simulink model "FingerEAERCtrl"  (R2012b)
settings: Solver=ode3  StartTime=0.0  StopTime=inf  FixedStep=.001  RelTol=1e-3
PreLoadFcn:
  | settupFilter;
InitFcn:
  | settupFilter;
values from neighbouring files (symbols this model uses):
  x0low = (eye(size(Alow))-Alow)\Blow*0    [settupFilter.m]
undefined symbols (not defined in the file or in its folder): Alow, Blow, Clow, Dlow
libraries: xpcnilib x4, xpclib x4, simulink x2
(part 1 of 2)
settings Model: SimulationMode=external  BufferReuse=off  Creator=Admin  LastModifiedBy=Admin
settings OptimizationCC: BlockReduction=off  OptimizeBlockIOStorage=off  BufferReuse=off  ExpressionFolding=off  LocalBlockOutputs=off
settings HardwareCC: ProdIntDivRoundTo=Zero  ProdEndianess=LittleEndian  ProdHWDeviceType=Generic->32-bit x86 compatible
settings RTWCC: SystemTargetFile=xpctarget.tlc  TemplateMakefile=xpc_default_tmf  Description=xPC Target  ProcessScript=xpctarget_make_rtw_hook  RTWCompilerOptimization=On
settings xpcTargetCC: TargetFcnLib=ansi_tfl_table_tmw.mat  CodeReplacementLibrary=XPC_BLAS  ParMdlRefBuildCompliant=on  ConcurrentExecutionCompliant=on  CombineSignalStateStructs=off  GRTInterface=on  xPCTaskExecutionProfile=off  xPCRL32EventNumber=5000  xPCLoadParamSetFile=off  xPCConcurrentTasks=off  xPCEnableSFAnimation=off

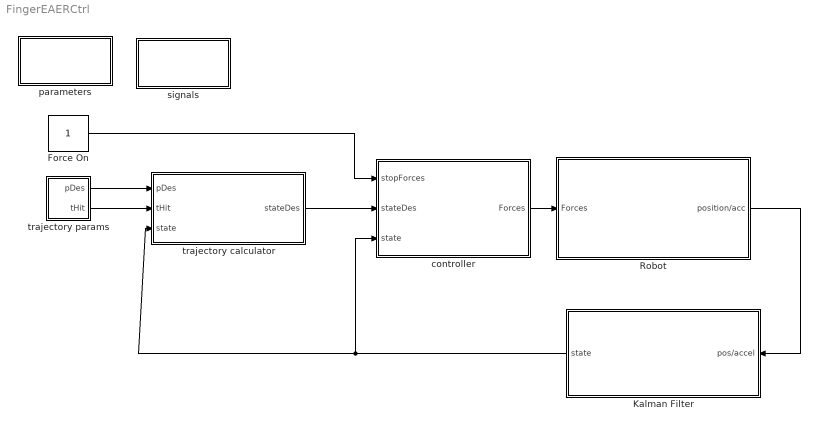
== system FingerEAERCtrl ==
  Force On : Constant
  Kalman Filter : Subsystem
  Robot : Subsystem
  controller : Subsystem
  parameters : Subsystem
  signals : Subsystem
  trajectory calculator : Subsystem
  trajectory params : Subsystem
  wires:
  Robot/1(position/acc) -> Kalman Filter/1(pos/accel)
  trajectory calculator/1(stateDes) -> controller/2(stateDes)
  controller/1(Forces) -> Robot/1(Forces)
  Kalman Filter/1(state) -> trajectory calculator/3(state), controller/3(state)
  trajectory params/1(pDes) -> trajectory calculator/1(pDes)
  trajectory params/2(tHit) -> trajectory calculator/2(tHit)
  Force On/1 -> controller/1(stopForces)

== system FingerEAERCtrl/Kalman Filter ==
  pos/accel : Inport
  Demux : Demux
  Mux : Mux  Inputs=2
  kalman1 : Subsystem
  kalman2 : Subsystem
  state : Outport
  tag scope: SIG_STATE=global
  wires:
  Demux/1 -> kalman1/1(position)
  Demux/2 -> kalman2/1(position)
  Demux/3 -> kalman1/2(acc)
  Demux/4 -> kalman2/2(acc)
  pos/accel/1 -> Demux/1
  kalman1/1(position/est_vel) -> Mux/1
  kalman2/1(position/est_vel) -> Mux/2
  Mux/1 -> [SIG_STATE], state/1

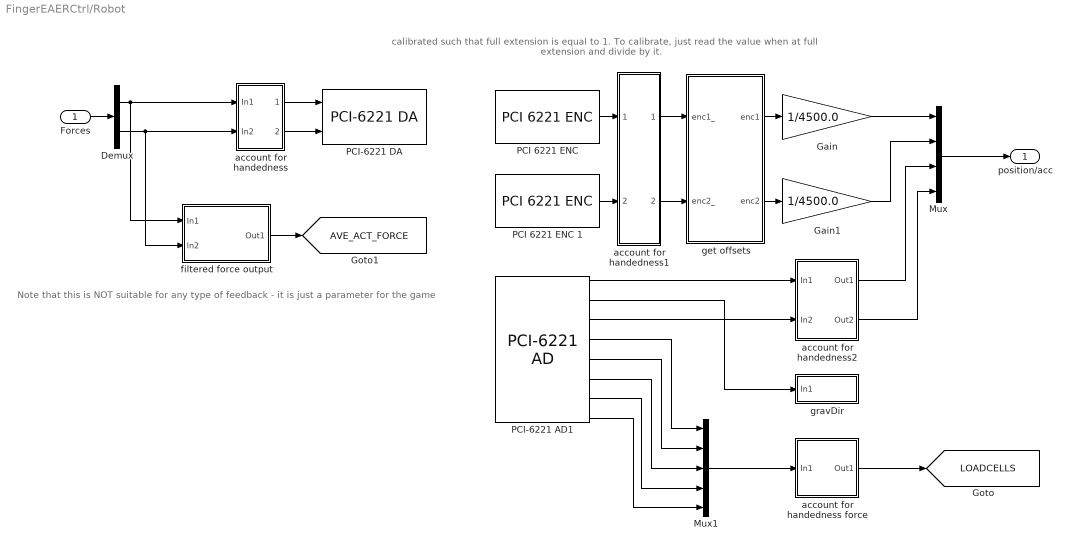
== system FingerEAERCtrl/Robot ==
  note: Note that this is NOT suitable for any type
      | of feedback - it is just a parameter for the game
  note: calibrated such that full extension is equal to 1. To calibrate, just read the value when at full extension and divide by it.
  Forces : Inport
  Demux : Demux  Outputs=2
  Gain : Gain  Gain=1/4500.0
  Gain1 : Gain  Gain=1/4500.0
  Mux : Mux
  Mux1 : Mux  Inputs=5
  "PCI 6221 ENC " : xpcnilib/Incremental Encoder/PCI 6221 ENC   channel=0  countMode=Quadrature Mode x4  initCount=0  reload=off  indexPhase=A low B low  filter=Minimum pulse width 125 nanoseconds  sampleTime=0.001  slot=-1
  PCI 6221 ENC 1 : xpcnilib/Incremental Encoder/PCI 6221 ENC   channel=1  countMode=Quadrature Mode x4  initCount=0  reload=off  indexPhase=A low B low  filter=Minimum pulse width 125 nanoseconds  sampleTime=0.001  slot=-1
  PCI-6221 AD1 : xpcnilib/A//D/M Series/PCI-6221 AD  channel=[1 2 3 4 5 6 7 8]  range=[10]  coupling=[0]  scantime=5e-6  sampletime=0.001  slot=-1
  PCI-6221 DA : xpcnilib/D//A/M Series/PCI-6221 DA  channel=[1 2]  reset=[1]  initValue=[0]  sampletime=0.001  slot=-1
  account for handedness : Subsystem
  account for handedness force : Subsystem
  account for handedness1 : Subsystem
  account for handedness2 : Subsystem
  filtered force output : Subsystem
  get offsets : Subsystem
  gravDir : Subsystem
  position/acc : Outport
  tag scope: AVE_ACT_FORCE=global, LOADCELLS=global
  wires:
  Gain/1 -> Mux/1
  Mux/1 -> position/acc/1
  Forces/1 -> Demux/1
  Gain1/1 -> Mux/2
  get offsets/1(enc1) -> Gain/1
  get offsets/2(enc2) -> Gain1/1
  Demux/1 -> filtered force output/1(In1), account for handedness/1(In1)
  Demux/2 -> filtered force output/2(In2), account for handedness/2(In2)
  account for handedness/2(Out2) -> PCI-6221 DA/2
  account for handedness/1(Out1) -> PCI-6221 DA/1
  "PCI 6221 ENC "/1 -> account for handedness1/1(In1)
  account for handedness1/1(Out1) -> get offsets/1(enc1_)
  account for handedness1/2(Out2) -> get offsets/2(enc2_)
  PCI 6221 ENC 1/1 -> account for handedness1/2(In2)
  PCI-6221 AD1/1 -> account for handedness2/1(In1)
  PCI-6221 AD1/3 -> account for handedness2/2(In2)
  account for handedness2/1(Out1) -> Mux/3
  account for handedness2/2(Out2) -> Mux/4
  PCI-6221 AD1/4 -> Mux1/1
  PCI-6221 AD1/5 -> Mux1/2
  PCI-6221 AD1/6 -> Mux1/3
  PCI-6221 AD1/7 -> Mux1/4
  PCI-6221 AD1/8 -> Mux1/5
  Mux1/1 -> account for handedness force/1(In1)
  account for handedness force/1(Out1) -> [LOADCELLS]
  PCI-6221 AD1/2 -> gravDir/1(In1)
  filtered force output/1(Out1) -> [AVE_ACT_FORCE]

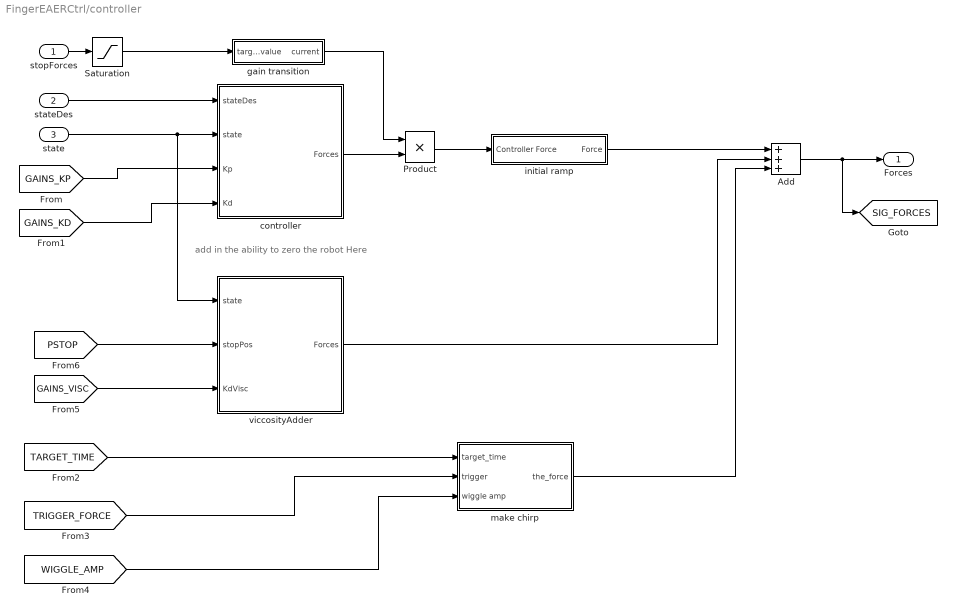
== system FingerEAERCtrl/controller ==
  note: add in the ability to zero the robot Here
  stopForces : Inport
  stateDes : Inport  Port=2
  state : Inport  Port=3
  Add : Sum  Inputs=+++
  Product : Product  RndMeth=Zero
  Saturation : Saturate  UpperLimit=1  LowerLimit=0
  controller : MATLAB Function  TreatAsAtomicUnit=on
  gain transition : Subsystem
  initial ramp : Subsystem
  make chirp : Subsystem
  viccosityAdder : MATLAB Function  TreatAsAtomicUnit=on
  Forces : Outport
  tag scope: SIG_FORCES=global
  wires:
  state/1 -> viccosityAdder/1(state), controller/2(state)
  [GAINS_KD] -> controller/4(Kd)
  [GAINS_KP] -> controller/3(Kp)
  stateDes/1 -> controller/1(stateDes)
  stopForces/1 -> Saturation/1
  Saturation/1 -> gain transition/1(target_value)
  controller/1(Forces) -> Product/2
  gain transition/1(current) -> Product/1
  Product/1 -> initial ramp/1(Controller Force)
  initial ramp/1(Force) -> Add/1
  Add/1 -> [SIG_FORCES], Forces/1
  [TARGET_TIME] -> make chirp/1(target_time)
  [TRIGGER_FORCE] -> make chirp/2(trigger)
  make chirp/1(the_force) -> Add/3
  [WIGGLE_AMP] -> make chirp/3(wiggle amp)
  viccosityAdder/1(Forces) -> Add/2
  [GAINS_VISC] -> viccosityAdder/3(KdVisc)
  [PSTOP] -> viccosityAdder/2(stopPos)

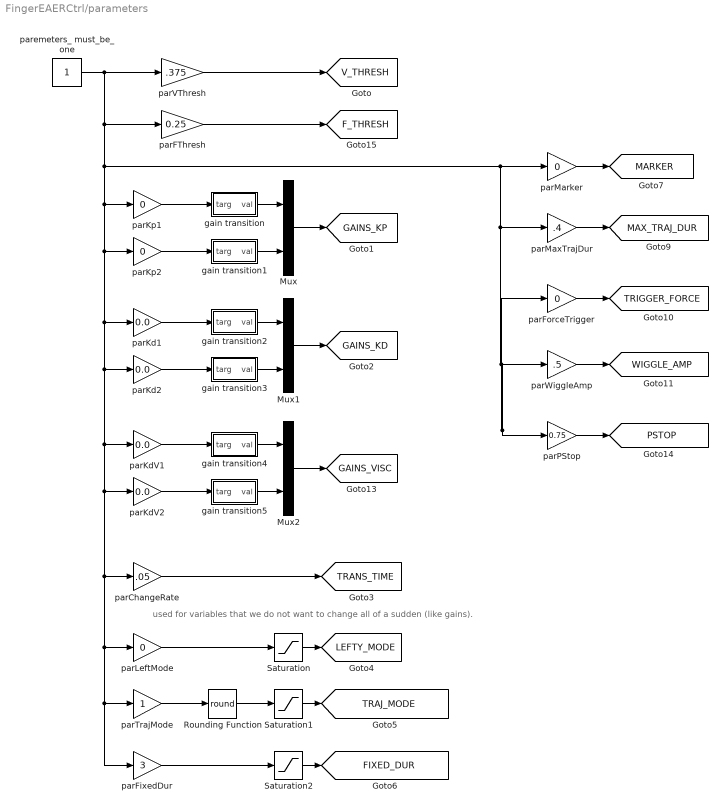
== system FingerEAERCtrl/parameters ==
  note: used for variables that we do not want to change all of a sudden (like gains).
  Mux : Mux  Inputs=2
  Mux1 : Mux  Inputs=2
  Mux2 : Mux  Inputs=2
  Rounding Function : Rounding  Operator=round
  Saturation : Saturate  UpperLimit=1  LowerLimit=0
  Saturation1 : Saturate  UpperLimit=4  LowerLimit=1
  Saturation2 : Saturate  UpperLimit=10  LowerLimit=.25
  gain transition : Subsystem
  gain transition1 : Subsystem
  gain transition2 : Subsystem
  gain transition3 : Subsystem
  gain transition4 : Subsystem
  gain transition5 : Subsystem
  parChangeRate : Gain  Gain=.05
  parFThresh : Gain  Gain=0.25
  parFixedDur : Gain  Gain=3
  parForceTrigger : Gain  Gain=0
  parKd1 : Gain  Gain=0.0
  parKd2 : Gain  Gain=0.0
  parKdV1 : Gain  Gain=0.0
  parKdV2 : Gain  Gain=0.0
  parKp1 : Gain  Gain=0
  parKp2 : Gain  Gain=0
  parLeftMode : Gain  Gain=0
  parMarker : Gain  Gain=0
  parMaxTrajDur : Gain  Gain=.4
  parPStop : Gain  Gain=0.75
  parTrajMode : Gain
  parVThresh : Gain  Gain=.375
  parWiggleAmp : Gain  Gain=.5
  paremeters_ must_be_one : Constant
  tag scope: FIXED_DUR=global, F_THRESH=global, GAINS_KD=global, GAINS_KP=global, GAINS_VISC=global, LEFTY_MODE=global, MARKER=global, MAX_TRAJ_DUR=global, PSTOP=global, TRAJ_MODE=global, TRANS_TIME=global, TRIGGER_FORCE=global, V_THRESH=global, WIGGLE_AMP=global
  wires:
  Mux/1 -> [GAINS_KP]
  Mux1/1 -> [GAINS_KD]
  Saturation/1 -> [LEFTY_MODE]
  gain transition/1(val) -> Mux/1
  gain transition1/1(val) -> Mux/2
  gain transition2/1(val) -> Mux1/1
  gain transition3/1(val) -> Mux1/2
  parVThresh/1 -> [V_THRESH]
  parKp1/1 -> gain transition/1(targ)
  parKp2/1 -> gain transition1/1(targ)
  parKd1/1 -> gain transition2/1(targ)
  parKd2/1 -> gain transition3/1(targ)
  parChangeRate/1 -> [TRANS_TIME]
  parLeftMode/1 -> Saturation/1
  Saturation1/1 -> [TRAJ_MODE]
  parTrajMode/1 -> Rounding Function/1
  Saturation2/1 -> [FIXED_DUR]
  parFixedDur/1 -> Saturation2/1
  Rounding Function/1 -> Saturation1/1
  parMarker/1 -> [MARKER]
  parMaxTrajDur/1 -> [MAX_TRAJ_DUR]
  parForceTrigger/1 -> [TRIGGER_FORCE]
  parWiggleAmp/1 -> [WIGGLE_AMP]
  Mux2/1 -> [GAINS_VISC]
  gain transition4/1(val) -> Mux2/1
  gain transition5/1(val) -> Mux2/2
  parKdV1/1 -> gain transition4/1(targ)
  parKdV2/1 -> gain transition5/1(targ)
  paremeters_ must_be_one/1 -> parVThresh/1, parFThresh/1, parKp1/1, parKp2/1, parKd1/1, parKd2/1, parKdV1/1, parKdV2/1, parChangeRate/1, parLeftMode/1, parFixedDur/1, parTrajMode/1, parPStop/1, parWiggleAmp/1, parForceTrigger/1, parMaxTrajDur/1, parMarker/1
  parPStop/1 -> [PSTOP]
  parFThresh/1 -> [F_THRESH]

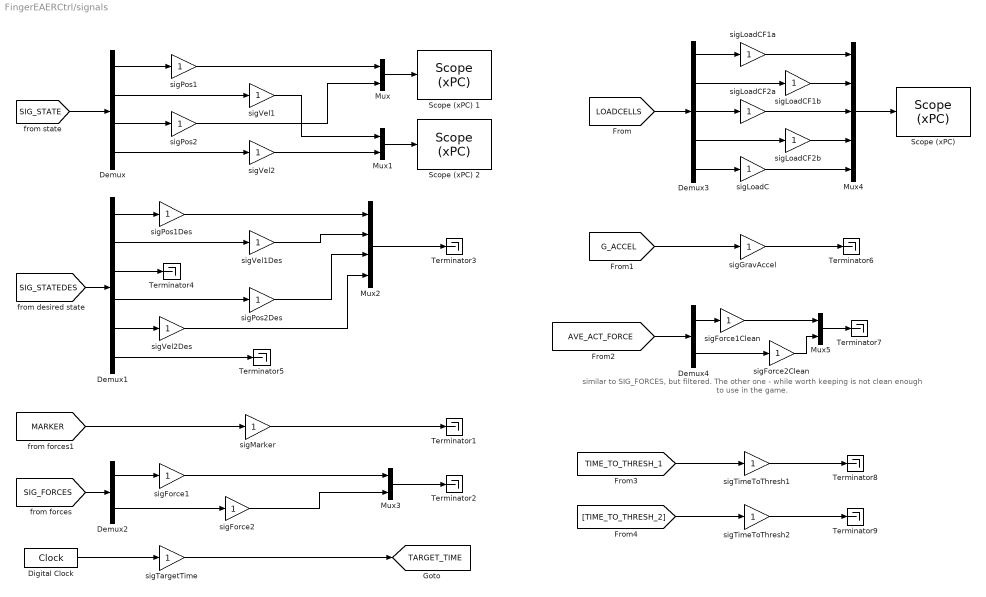
== system FingerEAERCtrl/signals ==
  note: similar to SIG_FORCES, but filtered. The other one - while worth keeping is not clean enough to use in the game.
  Demux : Demux
  Demux1 : Demux  Outputs=6
  Demux2 : Demux  Outputs=2
  Demux3 : Demux  Outputs=5
  Demux4 : Demux  Outputs=2
  Digital Clock : DigitalClock  SampleTime=.001
  Mux{,1,3,5} (4 alike) : Mux  Inputs=2
  Mux2 : Mux
  Mux4 : Mux  Inputs=5
  "Scope (xPC) " : xpclib/Misc./Scope (xPC)   scopeno=5  scopetype=Target  autostart=on  viewmode=Graphical redraw  formatstr='%15.6f'  grid=on  ylimits=[-3,3]  nosamples=500  noprepostsamples=0  interleave=1  triggermode=FreeRun  triggersignal=1  triggerlevel=0.0  triggerslope=Either  triggerscope=1  triggersample=0  filename=data.dat  mode=Lazy  writesize=512  autorestart=off  dynamicfilemode=off  maxwritefilesize=512*1024^2
  Scope (xPC) 1 : xpclib/Misc./Scope (xPC)   scopeno=1  scopetype=Target  autostart=on  viewmode=Graphical redraw  formatstr='%15.6f'  grid=on  ylimits=[0,1.1]  nosamples=500  noprepostsamples=0  interleave=1  triggermode=FreeRun  triggersignal=1  triggerlevel=0.0  triggerslope=Either  triggerscope=1  triggersample=0  filename=data.dat  mode=Lazy  writesize=512  autorestart=off  dynamicfilemode=off  maxwritefilesize=512*1024^2
  Scope (xPC) 2 : xpclib/Misc./Scope (xPC)   scopeno=2  scopetype=Target  autostart=on  viewmode=Graphical redraw  formatstr='%15.6f'  grid=on  ylimits=[-10,10]  nosamples=500  noprepostsamples=0  interleave=1  triggermode=FreeRun  triggersignal=1  triggerlevel=0.0  triggerslope=Either  triggerscope=1  triggersample=0  filename=data.dat  mode=Lazy  writesize=512  autorestart=off  dynamicfilemode=off  maxwritefilesize=512*1024^2
  Terminator{1..9} (9 alike) : Terminator
  sigForce1 : Gain
  sigForce1Clean : Gain
  sigForce2 : Gain
  sigForce2Clean : Gain
  sigGravAccel : Gain
  sigLoadC : Gain
  sigLoadCF1a : Gain
  sigLoadCF1b : Gain
  sigLoadCF2a : Gain
  sigLoadCF2b : Gain
  sigMarker : Gain
  sigPos1 : Gain
  sigPos1Des : Gain
  sigPos2 : Gain
  sigPos2Des : Gain
  sigTargetTime : Gain
  sigTimeToThresh1 : Gain
  sigTimeToThresh2 : Gain
  sigVel1 : Gain
  sigVel1Des : Gain
  sigVel2 : Gain
  sigVel2Des : Gain
  tag scope: TARGET_TIME=global
  wires:
  [SIG_STATE] -> Demux/1
  Demux/1 -> sigPos1/1
  Demux/2 -> sigVel1/1
  Demux/3 -> sigPos2/1
  Demux/4 -> sigVel2/1
  [SIG_STATEDES] -> Demux1/1
  Demux1/1 -> sigPos1Des/1
  Demux1/2 -> sigVel1Des/1
  Demux1/3 -> Terminator4/1
  Demux1/4 -> sigPos2Des/1
  Demux1/5 -> sigVel2Des/1
  Demux1/6 -> Terminator5/1
  Mux/1 -> Scope (xPC) 1/1
  Mux1/1 -> Scope (xPC) 2/1
  sigPos1/1 -> Mux/1
  sigPos2/1 -> Mux/2
  sigVel1/1 -> Mux1/1
  sigVel2/1 -> Mux1/2
  sigPos1Des/1 -> Mux2/1
  sigVel1Des/1 -> Mux2/2
  sigPos2Des/1 -> Mux2/3
  sigVel2Des/1 -> Mux2/4
  Mux2/1 -> Terminator3/1
  [SIG_FORCES] -> Demux2/1
  Demux2/1 -> sigForce1/1
  Demux2/2 -> sigForce2/1
  Mux3/1 -> Terminator2/1
  sigForce1/1 -> Mux3/1
  sigForce2/1 -> Mux3/2
  Digital Clock/1 -> sigTargetTime/1
  sigTargetTime/1 -> [TARGET_TIME]
  [MARKER] -> sigMarker/1
  sigMarker/1 -> Terminator1/1
  [LOADCELLS] -> Demux3/1
  Demux3/1 -> sigLoadCF1a/1
  Demux3/2 -> sigLoadCF1b/1
  Demux3/3 -> sigLoadCF2a/1
  Demux3/4 -> sigLoadCF2b/1
  Demux3/5 -> sigLoadC/1
  sigLoadCF1a/1 -> Mux4/1
  sigLoadCF1b/1 -> Mux4/2
  sigLoadCF2a/1 -> Mux4/3
  sigLoadCF2b/1 -> Mux4/4
  sigLoadC/1 -> Mux4/5
  Mux4/1 -> "Scope (xPC) "/1
  [G_ACCEL] -> sigGravAccel/1
  sigGravAccel/1 -> Terminator6/1
  [AVE_ACT_FORCE] -> Demux4/1
  Demux4/1 -> sigForce1Clean/1
  Demux4/2 -> sigForce2Clean/1
  Mux5/1 -> Terminator7/1
  sigForce1Clean/1 -> Mux5/1
  sigForce2Clean/1 -> Mux5/2
  sigTimeToThresh1/1 -> Terminator8/1
  [TIME_TO_THRESH_1] -> sigTimeToThresh1/1
  sigTimeToThresh2/1 -> Terminator9/1
  [TIME_TO_THRESH_2] -> sigTimeToThresh2/1

== system FingerEAERCtrl/trajectory calculator ==
  pDes : Inport
  tHit : Inport  Port=2
  state : Inport  Port=3
  Multiport Switch : MultiPortSwitch  Inputs=4
  mode 1: sub-init : Subsystem
  mode 2: auto initiated : Subsystem
  mode 3: auto init no return : Subsystem
  mode 4: sub init no return : Subsystem
  stateDes : Outport
  tag scope: SIG_STATEDES=global
  wires:
  pDes/1 -> mode 4: sub init no return/1(pDes), mode 3: auto init no return/1(pDes), mode 2: auto initiated/1(pDes), mode 1: sub-init/1(pDes)
  state/1 -> mode 1: sub-init/3(state), mode 4: sub init no return/3(state), mode 3: auto init no return/3(state), mode 2: auto initiated/3(state)
  mode 1: sub-init/1(trajectory) -> Multiport Switch/2
  mode 2: auto initiated/1(trajectory) -> Multiport Switch/3
  mode 3: auto init no return/1(trajectory) -> Multiport Switch/4
  [TRAJ_MODE] -> Multiport Switch/1
  mode 4: sub init no return/1(trajectory) -> Multiport Switch/5
  Multiport Switch/1 -> [SIG_STATEDES], stateDes/1
  tHit/1 -> mode 4: sub init no return/2(tHit), mode 3: auto init no return/2(tHit), mode 2: auto initiated/2(tHit), mode 1: sub-init/2(tHit)

== system FingerEAERCtrl/trajectory params ==
  Mux : Mux  Inputs=2
  Mux1 : Mux  Inputs=2
  parP1Des : Gain  Gain=.95
  parP2Des : Gain  Gain=.95
  parTHit1 : Gain  Gain=50
  parTHit2 : Gain  Gain=40
  unity_traj : Constant
  pDes : Outport
  tHit : Outport  Port=2
  wires:
  Mux/1 -> pDes/1
  Mux1/1 -> tHit/1
  parP1Des/1 -> Mux/1
  parP2Des/1 -> Mux/2
  parTHit1/1 -> Mux1/1
  parTHit2/1 -> Mux1/2
  unity_traj/1 -> parTHit2/1, parTHit1/1, parP2Des/1, parP1Des/1

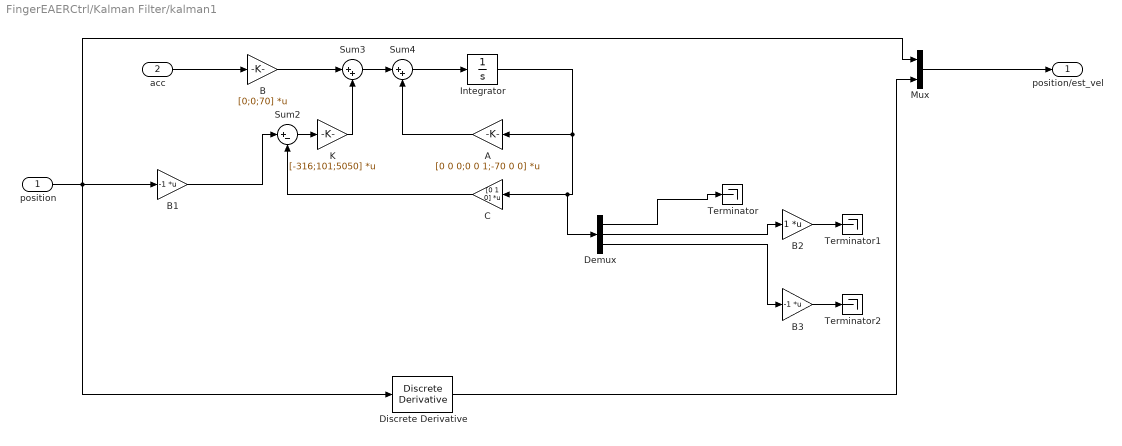
== system FingerEAERCtrl/Kalman Filter/kalman1 ==
  position : Inport
  acc : Inport  Port=2
  A : Gain  Gain=[0 0 0;0 0 1;-70 0 0]  Multiplication=Matrix(K*u)
  B : Gain  Gain=[0;0;70]  Multiplication=Matrix(K*u)
  B1 : Gain  Gain=-1  Multiplication=Matrix(K*u)
  B2 : Gain  Multiplication=Matrix(K*u)
  B3 : Gain  Gain=-1  Multiplication=Matrix(K*u)
  C : Gain  Gain=[0 1 0]  Multiplication=Matrix(K*u)
  Demux : Demux  Outputs=3
  Discrete Derivative : simulink/Discrete/Discrete Derivative  gainval=1.0  ICPrevScaledInput=0.0  InputProcessing=Inherited  OutMin=[]  OutMax=[]  OutDataType=fixdt(1, 16)  OutScaling=2^-10  DoSatur=off
  Integrator : Integrator  InitialCondition=[1.5;0;0]
  K : Gain  Gain=[-316;101;5050]  Multiplication=Matrix(K*u)
  Mux : Mux  Inputs=2
  Sum2 : Sum  Inputs=|+-
  Sum3 : Sum  Inputs=|++
  Sum4 : Sum  Inputs=|++
  Terminator : Terminator
  Terminator1 : Terminator
  Terminator2 : Terminator
  position/est_vel : Outport
  wires:
  Integrator/1 -> A/1, C/1, Demux/1
  C/1 -> Sum2/2
  Sum2/1 -> K/1
  B/1 -> Sum3/1
  K/1 -> Sum3/2
  Sum3/1 -> Sum4/1
  A/1 -> Sum4/2
  Sum4/1 -> Integrator/1
  Demux/2 -> B2/1
  Demux/3 -> B3/1
  Demux/1 -> Terminator/1
  B1/1 -> Sum2/1
  B2/1 -> Terminator1/1
  Mux/1 -> position/est_vel/1
  acc/1 -> B/1
  position/1 -> Discrete Derivative/1, Mux/1, B1/1
  Discrete Derivative/1 -> Mux/2
  B3/1 -> Terminator2/1

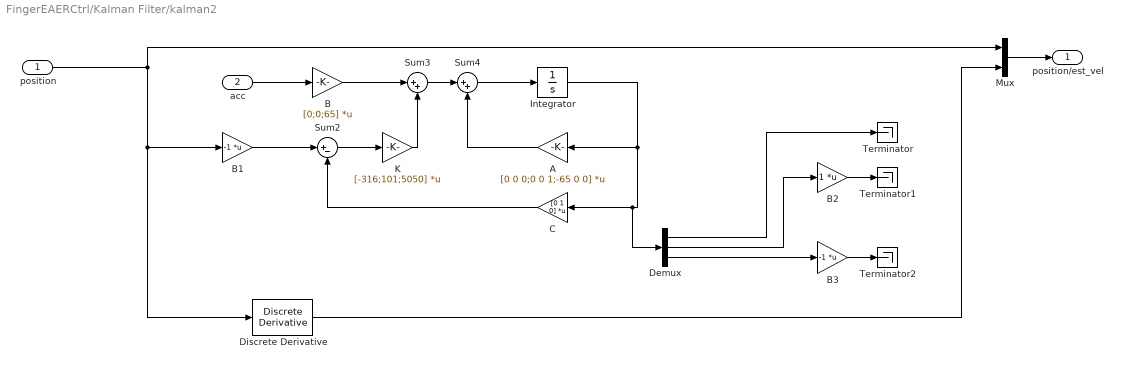
== system FingerEAERCtrl/Kalman Filter/kalman2 ==
  position : Inport
  acc : Inport  Port=2
  A : Gain  Gain=[0 0 0;0 0 1;-65 0 0]  Multiplication=Matrix(K*u)
  B : Gain  Gain=[0;0;65]  Multiplication=Matrix(K*u)
  B1 : Gain  Gain=-1  Multiplication=Matrix(K*u)
  B2 : Gain  Multiplication=Matrix(K*u)
  B3 : Gain  Gain=-1  Multiplication=Matrix(K*u)
  C : Gain  Gain=[0 1 0]  Multiplication=Matrix(K*u)
  Demux : Demux  Outputs=3
  Discrete Derivative : simulink/Discrete/Discrete Derivative  gainval=1.0  ICPrevScaledInput=0.0  InputProcessing=Inherited  OutMin=[]  OutMax=[]  OutDataType=fixdt(1, 16)  OutScaling=2^-10  DoSatur=off
  Integrator : Integrator  InitialCondition=[1.5;0;0]
  K : Gain  Gain=[-316;101;5050]  Multiplication=Matrix(K*u)
  Mux : Mux  Inputs=2
  Sum2 : Sum  Inputs=|+-
  Sum3 : Sum  Inputs=|++
  Sum4 : Sum  Inputs=|++
  Terminator : Terminator
  Terminator1 : Terminator
  Terminator2 : Terminator
  position/est_vel : Outport
  wires:
  acc/1 -> B/1
  Mux/1 -> position/est_vel/1
  B2/1 -> Terminator1/1
  B1/1 -> Sum2/1
  Demux/1 -> Terminator/1
  Demux/3 -> B3/1
  Demux/2 -> B2/1
  Sum4/1 -> Integrator/1
  A/1 -> Sum4/2
  Sum3/1 -> Sum4/1
  K/1 -> Sum3/2
  B/1 -> Sum3/1
  Sum2/1 -> K/1
  C/1 -> Sum2/2
  Integrator/1 -> Demux/1, C/1, A/1
  position/1 -> Discrete Derivative/1, B1/1, Mux/1
  Discrete Derivative/1 -> Mux/2
  B3/1 -> Terminator2/1

== system FingerEAERCtrl/Robot/account for handedness ==
  In1 : Inport
  In2 : Inport  Port=2
  MATLAB Function : MATLAB Function  TreatAsAtomicUnit=on
  Out1 : Outport
  Out2 : Outport  Port=2
  wires:
  MATLAB Function/1(output1) -> Out1/1
  MATLAB Function/2(output2) -> Out2/1
  In1/1 -> MATLAB Function/1(input1)
  In2/1 -> MATLAB Function/2(input2)
  [LEFTY_MODE] -> MATLAB Function/3(leftyMode)

== system FingerEAERCtrl/Robot/account for handedness force ==
  In1 : Inport
  MATLAB Function : MATLAB Function  TreatAsAtomicUnit=on
  Out1 : Outport
  wires:
  [LEFTY_MODE] -> MATLAB Function/2(leftyMode)
  MATLAB Function/1(output) -> Out1/1
  In1/1 -> MATLAB Function/1(inp1)

== system FingerEAERCtrl/Robot/account for handedness1 ==
  In1 : Inport
  In2 : Inport  Port=2
  MATLAB Function : MATLAB Function  TreatAsAtomicUnit=on
  Out1 : Outport
  Out2 : Outport  Port=2
  wires:
  MATLAB Function/1(output1) -> Out1/1
  MATLAB Function/2(output2) -> Out2/1
  In1/1 -> MATLAB Function/1(input1)
  In2/1 -> MATLAB Function/2(input2)
  [LEFTY_MODE] -> MATLAB Function/3(leftyMode)

== system FingerEAERCtrl/Robot/account for handedness2 ==
  In1 : Inport
  In2 : Inport  Port=2
  MATLAB Function : MATLAB Function  TreatAsAtomicUnit=on
  Out1 : Outport
  Out2 : Outport  Port=2
  wires:
  MATLAB Function/1(output1) -> Out1/1
  MATLAB Function/2(output2) -> Out2/1
  In1/1 -> MATLAB Function/1(input1)
  In2/1 -> MATLAB Function/2(input2)
  [LEFTY_MODE] -> MATLAB Function/3(leftyMode)

== system FingerEAERCtrl/Robot/filtered force output ==
  In1 : Inport
  In2 : Inport  Port=2
  Low Pass 100 Hz : DiscreteStateSpace  A=Alow  B=Blow  C=Clow  D=Dlow  X0=x0low  SampleTime=-1
  Low Pass 100 Hz1 : DiscreteStateSpace  A=Alow  B=Blow  C=Clow  D=Dlow  X0=x0low  SampleTime=-1
  Memory : Memory
  Memory1 : Memory
  Mux2 : Mux  Inputs=2
  Out1 : Outport
  wires:
  Low Pass 100 Hz1/1 -> Memory1/1
  Low Pass 100 Hz/1 -> Memory/1
  Mux2/1 -> Out1/1
  In1/1 -> Low Pass 100 Hz/1
  In2/1 -> Low Pass 100 Hz1/1
  Memory/1 -> Mux2/1
  Memory1/1 -> Mux2/2

== system FingerEAERCtrl/Robot/get offsets ==
  enc1_ : Inport
  enc2_ : Inport  Port=2
  Digital Clock : DigitalClock  SampleTime=.001
  MATLAB Function : MATLAB Function  TreatAsAtomicUnit=on
  Memory : Memory
  Memory1 : Memory  X0=[0,0]
  enc1 : Outport
  enc2 : Outport  Port=2
  wires:
  Memory/1 -> MATLAB Function/5(nSamples_)
  Memory1/1 -> MATLAB Function/4(summedVals_)
  MATLAB Function/3(summedVals) -> Memory1/1
  Digital Clock/1 -> MATLAB Function/3(time)
  MATLAB Function/1(encoder1) -> enc1/1
  MATLAB Function/2(encoder2) -> enc2/1
  enc2_/1 -> MATLAB Function/2(enc2_)
  enc1_/1 -> MATLAB Function/1(enc1_)
  MATLAB Function/4(nSamples) -> Memory/1

== system FingerEAERCtrl/Robot/gravDir ==
  In1 : Inport
  Constant : Constant  Value=1.5
  Scope (xPC) 1 : xpclib/Misc./Scope (xPC)   scopeno=3  scopetype=Target  autostart=on  viewmode=Graphical redraw  formatstr='%15.6f'  grid=on  ylimits=[.03,.1]  nosamples=500  noprepostsamples=0  interleave=1  triggermode=FreeRun  triggersignal=1  triggerlevel=0.0  triggerslope=Either  triggerscope=1  triggersample=0  filename=data.dat  mode=Lazy  writesize=512  autorestart=off  dynamicfilemode=off  maxwritefilesize=512*1024^2
  Sum : Sum  Inputs=|+-
  gain : Gain  Gain=.172
  tag scope: G_ACCEL=global
  wires:
  gain/1 -> [G_ACCEL], Scope (xPC) 1/1
  Sum/1 -> gain/1
  Constant/1 -> Sum/2
  In1/1 -> Sum/1

== system FingerEAERCtrl/controller/gain transition ==
  target_value : Inport
  Memory : Memory  X0=zeros(1,4)
  gainramp : MATLAB Function  TreatAsAtomicUnit=on
  current : Outport
  wires:
  Memory/1 -> gainramp/3(state)
  gainramp/2(state1) -> Memory/1
  [TRANS_TIME] -> gainramp/1(tr)
  gainramp/1(val) -> current/1
  target_value/1 -> gainramp/2(valD)

== system FingerEAERCtrl/controller/initial ramp ==
  note: In the first five seconds of operation, have the actuators pull the fingers back so that the robot can zero itself accurately
  Controller Force : Inport
  MATLAB Function : MATLAB Function  TreatAsAtomicUnit=on
  Saturation1 : Saturate  UpperLimit=2.5  LowerLimit=-2.5
  ramp : MATLAB Function  TreatAsAtomicUnit=on
  Force : Outport
  wires:
  ramp/1(y) -> Saturation1/1
  Controller Force/1 -> MATLAB Function/1(ctrlForce)
  Saturation1/1 -> MATLAB Function/2(rampForce)
  [TARGET_TIME] -> MATLAB Function/3(time), ramp/1(tTime)
  MATLAB Function/1(Force) -> Force/1

== system FingerEAERCtrl/controller/make chirp ==
  target_time : Inport
  trigger : Inport  Port=2
  wiggle amp : Inport  Port=3
  MATLAB Function : MATLAB Function  TreatAsAtomicUnit=on
  MATLAB Function1 : MATLAB Function  TreatAsAtomicUnit=on
  Memory : Memory
  Memory1 : Memory
  Memory2 : Memory
  Mux : Mux  Inputs=2
  the_force : Outport
  wires:
  Memory/1 -> MATLAB Function1/2(oldTrigger)
  target_time/1 -> MATLAB Function/1(now)
  trigger/1 -> MATLAB Function1/1(trigger)
  MATLAB Function1/1(pulse) -> MATLAB Function/2(trigger)
  Mux/1 -> the_force/1
  MATLAB Function/3(tStart_) -> Memory2/1
  MATLAB Function/4(fNum_) -> Memory1/1
  Memory2/1 -> MATLAB Function/4(tStart)
  Memory1/1 -> MATLAB Function/5(fNum)
  MATLAB Function/2(f2) -> Mux/2
  MATLAB Function/1(f1) -> Mux/1
  MATLAB Function1/2(oldTrigger_) -> Memory/1
  wiggle amp/1 -> MATLAB Function/3(wiggleAmp)

== system FingerEAERCtrl/parameters/gain transition ==
  targ : Inport
  Memory : Memory  X0=zeros(1,4)
  gainramp : MATLAB Function  TreatAsAtomicUnit=on
  val : Outport
  wires:
  Memory/1 -> gainramp/3(state)
  gainramp/2(state1) -> Memory/1
  [TRANS_TIME] -> gainramp/1(tr)
  gainramp/1(val) -> val/1
  targ/1 -> gainramp/2(valD)

== system FingerEAERCtrl/parameters/gain transition1 ==
  targ : Inport
  Memory : Memory  X0=zeros(1,4)
  gainramp : MATLAB Function  TreatAsAtomicUnit=on
  val : Outport
  wires:
  Memory/1 -> gainramp/3(state)
  gainramp/2(state1) -> Memory/1
  [TRANS_TIME] -> gainramp/1(tr)
  gainramp/1(val) -> val/1
  targ/1 -> gainramp/2(valD)

== system FingerEAERCtrl/parameters/gain transition2 ==
  targ : Inport
  Memory : Memory  X0=zeros(1,4)
  gainramp : MATLAB Function  TreatAsAtomicUnit=on
  val : Outport
  wires:
  Memory/1 -> gainramp/3(state)
  gainramp/2(state1) -> Memory/1
  [TRANS_TIME] -> gainramp/1(tr)
  gainramp/1(val) -> val/1
  targ/1 -> gainramp/2(valD)

== system FingerEAERCtrl/parameters/gain transition3 ==
  targ : Inport
  Memory : Memory  X0=zeros(1,4)
  gainramp : MATLAB Function  TreatAsAtomicUnit=on
  val : Outport
  wires:
  Memory/1 -> gainramp/3(state)
  gainramp/2(state1) -> Memory/1
  [TRANS_TIME] -> gainramp/1(tr)
  gainramp/1(val) -> val/1
  targ/1 -> gainramp/2(valD)

== system FingerEAERCtrl/parameters/gain transition4 ==
  targ : Inport
  Memory : Memory  X0=zeros(1,4)
  gainramp : MATLAB Function  TreatAsAtomicUnit=on
  val : Outport
  wires:
  Memory/1 -> gainramp/3(state)
  gainramp/2(state1) -> Memory/1
  [TRANS_TIME] -> gainramp/1(tr)
  gainramp/1(val) -> val/1
  targ/1 -> gainramp/2(valD)

== system FingerEAERCtrl/parameters/gain transition5 ==
  targ : Inport
  Memory : Memory  X0=zeros(1,4)
  gainramp : MATLAB Function  TreatAsAtomicUnit=on
  val : Outport
  wires:
  Memory/1 -> gainramp/3(state)
  gainramp/2(state1) -> Memory/1
  [TRANS_TIME] -> gainramp/1(tr)
  gainramp/1(val) -> val/1
  targ/1 -> gainramp/2(valD)

== system FingerEAERCtrl/trajectory calculator/mode 1: sub-init ==
  pDes : Inport
  tHit : Inport  Port=2
  state : Inport  Port=3
  Demux : Demux  Outputs=2
  Demux1 : Demux  Outputs=2
  Demux2 : Demux
  Mux : Mux  Inputs=2
  get human force : Subsystem
  rt minimum jerk trajectory calc : Subsystem
  rt minimum jerk trajectory calc1 : Subsystem
  trajectory : Outport
  wires:
  pDes/1 -> Demux/1
  tHit/1 -> Demux1/1
  state/1 -> Demux2/1
  Demux/1 -> rt minimum jerk trajectory calc/1(Pdes)
  Demux1/1 -> rt minimum jerk trajectory calc/2(Tdes)
  Demux2/1 -> rt minimum jerk trajectory calc/3(pos)
  Demux2/2 -> rt minimum jerk trajectory calc/4(vel)
  Demux/2 -> rt minimum jerk trajectory calc1/1(Pdes)
  Demux1/2 -> rt minimum jerk trajectory calc1/2(Tdes)
  Demux2/3 -> rt minimum jerk trajectory calc1/3(pos)
  Demux2/4 -> rt minimum jerk trajectory calc1/4(vel)
  rt minimum jerk trajectory calc/1(trajectory) -> Mux/1
  rt minimum jerk trajectory calc1/1(trajectory) -> Mux/2
  Mux/1 -> trajectory/1
  [AVE_ACT_FORCE] -> get human force/1(forces)
  get human force/1(h_force1) -> rt minimum jerk trajectory calc/5(force)
  get human force/2(h_force2) -> rt minimum jerk trajectory calc1/5(force)

== system FingerEAERCtrl/trajectory calculator/mode 2: auto initiated ==
  note: the robot return the subjects to their starting position after the movement is complete
  note: the subjects do not need to tinitiate the movement.
  note: this version does moves the subjects automagically when the time is right
  pDes : Inport
  tHit : Inport  Port=2
  state : Inport  Port=3
  Demux : Demux  Outputs=2
  Demux1 : Demux  Outputs=2
  Demux2 : Demux
  Mux : Mux  Inputs=2
  rt minimum jerk trajectory : Subsystem
  rt minimum jerk trajectory1 : Subsystem
  trajectory : Outport
  wires:
  pDes/1 -> Demux/1
  tHit/1 -> Demux1/1
  state/1 -> Demux2/1
  Demux/1 -> rt minimum jerk trajectory/1(Pdes)
  Demux1/1 -> rt minimum jerk trajectory/2(Tdes)
  Demux2/1 -> rt minimum jerk trajectory/3(pos)
  Demux2/2 -> rt minimum jerk trajectory/4(vel)
  Demux/2 -> rt minimum jerk trajectory1/1(Pdes)
  Demux1/2 -> rt minimum jerk trajectory1/2(Tdes)
  Demux2/3 -> rt minimum jerk trajectory1/3(pos)
  Demux2/4 -> rt minimum jerk trajectory1/4(vel)
  rt minimum jerk trajectory/1(trajectory) -> Mux/1
  rt minimum jerk trajectory1/1(trajectory) -> Mux/2
  Mux/1 -> trajectory/1

== system FingerEAERCtrl/trajectory calculator/mode 3: auto init no return ==
  note: this is identical to the one above, but it will NOT return subjects to their starting position
  note: the subjects do not need to initiate the movement.
  note: this version does moves the subjects automagically when the time is right
  pDes : Inport
  tHit : Inport  Port=2
  state : Inport  Port=3
  Demux : Demux  Outputs=2
  Demux1 : Demux  Outputs=2
  Demux2 : Demux
  Mux : Mux  Inputs=2
  PosTerminator : Terminator
  PosTerminator1 : Terminator
  rt minimum jerk trajectory : Subsystem
  rt minimum jerk trajectory1 : Subsystem
  trajectory : Outport
  wires:
  pDes/1 -> Demux/1
  tHit/1 -> Demux1/1
  state/1 -> Demux2/1
  Demux/1 -> rt minimum jerk trajectory/1(Pdes)
  Demux1/1 -> rt minimum jerk trajectory/2(Tdes)
  Demux2/1 -> PosTerminator/1
  Demux2/2 -> rt minimum jerk trajectory/3(vel)
  Demux/2 -> rt minimum jerk trajectory1/1(Pdes)
  Demux1/2 -> rt minimum jerk trajectory1/2(Tdes)
  Demux2/3 -> PosTerminator1/1
  Demux2/4 -> rt minimum jerk trajectory1/3(vel)
  rt minimum jerk trajectory/1(trajectory) -> Mux/1
  rt minimum jerk trajectory1/1(trajectory) -> Mux/2
  Mux/1 -> trajectory/1

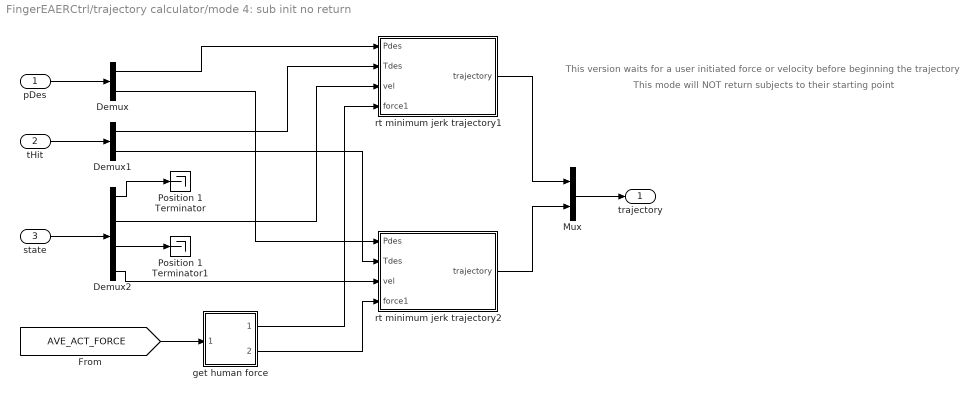
== system FingerEAERCtrl/trajectory calculator/mode 4: sub init no return ==
  note: This mode will NOT return subjects to their starting point
  note: This version waits for a user initiated force or velocity before beginning the trajectory
  pDes : Inport
  tHit : Inport  Port=2
  state : Inport  Port=3
  Demux : Demux  Outputs=2
  Demux1 : Demux  Outputs=2
  Demux2 : Demux
  Mux : Mux  Inputs=2
  Position 1 Terminator : Terminator
  Position 1 Terminator1 : Terminator
  get human force : Subsystem
  rt minimum jerk trajectory1 : Subsystem
  rt minimum jerk trajectory2 : Subsystem
  trajectory : Outport
  wires:
  pDes/1 -> Demux/1
  tHit/1 -> Demux1/1
  state/1 -> Demux2/1
  Demux/1 -> rt minimum jerk trajectory1/1(Pdes)
  Demux1/1 -> rt minimum jerk trajectory1/2(Tdes)
  Demux2/1 -> Position 1 Terminator/1
  Demux2/2 -> rt minimum jerk trajectory1/3(vel)
  Demux/2 -> rt minimum jerk trajectory2/1(Pdes)
  Demux1/2 -> rt minimum jerk trajectory2/2(Tdes)
  Demux2/3 -> Position 1 Terminator1/1
  Demux2/4 -> rt minimum jerk trajectory2/3(vel)
  rt minimum jerk trajectory1/1(trajectory) -> Mux/1
  Mux/1 -> trajectory/1
  [AVE_ACT_FORCE] -> get human force/1(forces)
  get human force/1(h_force1) -> rt minimum jerk trajectory1/4(force1)
  get human force/2(h_force2) -> rt minimum jerk trajectory2/4(force1)
  rt minimum jerk trajectory2/1(trajectory) -> Mux/2

== system FingerEAERCtrl/trajectory calculator/mode 1: sub-init/get human force ==
  note: flip robot force to get human force
  forces : Inport
  Constant : Constant  Value=-1
  Demux3 : Demux  Outputs=2
  Product : Product  RndMeth=Zero
  Product1 : Product  RndMeth=Zero
  h_force1 : Outport
  h_force2 : Outport  Port=2
  wires:
  forces/1 -> Demux3/1
  Constant/1 -> Product1/2, Product/2
  Product/1 -> h_force1/1
  Demux3/1 -> Product/1
  Demux3/2 -> Product1/1
  Product1/1 -> h_force2/1

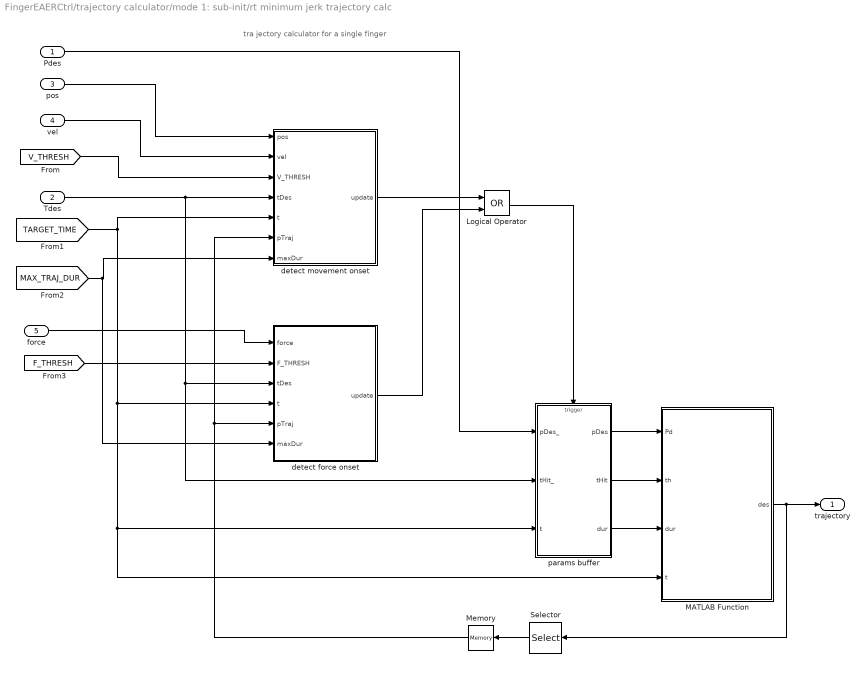
== system FingerEAERCtrl/trajectory calculator/mode 1: sub-init/rt minimum jerk trajectory calc ==
  note: tra jectory calculator for a single finger
  Pdes : Inport
  Tdes : Inport  Port=2
  pos : Inport  Port=3
  vel : Inport  Port=4
  force : Inport  Port=5
  Logical Operator : Logic  Operator=OR  AllPortsSameDT=off  OutDataTypeStr=boolean
  MATLAB Function : MATLAB Function  TreatAsAtomicUnit=on
  Memory : Memory
  Selector : Selector  InputPortWidth=3  IndexOptions=Index vector (dialog)  Indices=[1]  OutputSizes=1
  detect force onset : MATLAB Function  TreatAsAtomicUnit=on
  detect movement onset : MATLAB Function  TreatAsAtomicUnit=on
  params buffer : Subsystem
  trajectory : Outport
  wires:
  [TARGET_TIME] -> detect force onset/4(t), MATLAB Function/4(t), params buffer/3(t), detect movement onset/5(t)
  vel/1 -> detect movement onset/2(vel)
  [V_THRESH] -> detect movement onset/3(V_THRESH)
  Tdes/1 -> detect movement onset/4(tDes), detect force onset/3(tDes), params buffer/2(tHit_)
  Pdes/1 -> params buffer/1(pDes_)
  params buffer/1(pDes) -> MATLAB Function/1(Pd)
  params buffer/2(tHit) -> MATLAB Function/2(th)
  params buffer/3(dur) -> MATLAB Function/3(dur)
  MATLAB Function/1(des) -> Selector/1, trajectory/1
  pos/1 -> detect movement onset/1(pos)
  Selector/1 -> Memory/1
  Memory/1 -> detect force onset/5(pTraj), detect movement onset/6(pTraj)
  [MAX_TRAJ_DUR] -> detect force onset/6(maxDur), detect movement onset/7(maxDur)
  [F_THRESH] -> detect force onset/2(F_THRESH)
  detect movement onset/1(update) -> Logical Operator/1
  detect force onset/1(update) -> Logical Operator/2
  Logical Operator/1 -> params buffer/Trigger
  force/1 -> detect force onset/1(force)

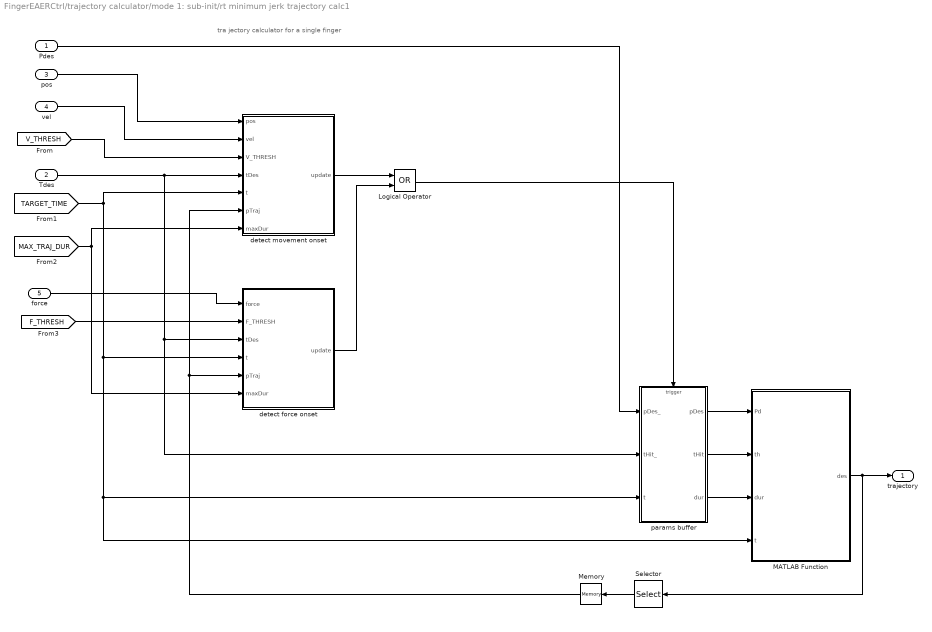
== system FingerEAERCtrl/trajectory calculator/mode 1: sub-init/rt minimum jerk trajectory calc1 ==
  note: tra jectory calculator for a single finger
  Pdes : Inport
  Tdes : Inport  Port=2
  pos : Inport  Port=3
  vel : Inport  Port=4
  force : Inport  Port=5
  Logical Operator : Logic  Operator=OR  AllPortsSameDT=off  OutDataTypeStr=boolean
  MATLAB Function : MATLAB Function  TreatAsAtomicUnit=on
  Memory : Memory
  Selector : Selector  InputPortWidth=3  IndexOptions=Index vector (dialog)  Indices=[1]  OutputSizes=1
  detect force onset : MATLAB Function  TreatAsAtomicUnit=on
  detect movement onset : MATLAB Function  TreatAsAtomicUnit=on
  params buffer : Subsystem
  trajectory : Outport
  wires:
  [TARGET_TIME] -> detect force onset/4(t), MATLAB Function/4(t), params buffer/3(t), detect movement onset/5(t)
  vel/1 -> detect movement onset/2(vel)
  [V_THRESH] -> detect movement onset/3(V_THRESH)
  Tdes/1 -> detect movement onset/4(tDes), detect force onset/3(tDes), params buffer/2(tHit_)
  Pdes/1 -> params buffer/1(pDes_)
  params buffer/1(pDes) -> MATLAB Function/1(Pd)
  params buffer/2(tHit) -> MATLAB Function/2(th)
  params buffer/3(dur) -> MATLAB Function/3(dur)
  MATLAB Function/1(des) -> Selector/1, trajectory/1
  pos/1 -> detect movement onset/1(pos)
  Selector/1 -> Memory/1
  Memory/1 -> detect force onset/5(pTraj), detect movement onset/6(pTraj)
  [MAX_TRAJ_DUR] -> detect force onset/6(maxDur), detect movement onset/7(maxDur)
  [F_THRESH] -> detect force onset/2(F_THRESH)
  force/1 -> detect force onset/1(force)
  detect movement onset/1(update) -> Logical Operator/1
  detect force onset/1(update) -> Logical Operator/2
  Logical Operator/1 -> params buffer/Trigger

== system FingerEAERCtrl/trajectory calculator/mode 2: auto initiated/rt minimum jerk trajectory ==
  note: tra jectory calculator for a single finger
  Pdes : Inport
  Tdes : Inport  Port=2
  pos : Inport  Port=3
  vel : Inport  Port=4
  MATLAB Function : MATLAB Function  TreatAsAtomicUnit=on
  Terminator : Terminator
  detect change : Subsystem
  params buffer : Subsystem
  trajectory : Outport
  wires:
  [TARGET_TIME] -> params buffer/4(t), MATLAB Function/5(t)
  Tdes/1 -> detect change/1(pDes), params buffer/3(tHit_)
  Pdes/1 -> params buffer/1(pDes_)
  params buffer/1(pDes) -> MATLAB Function/1(Pd)
  params buffer/3(tHit) -> MATLAB Function/3(th)
  params buffer/4(dur) -> MATLAB Function/4(dur)
  MATLAB Function/1(des) -> trajectory/1
  [FIXED_DUR] -> params buffer/5(fixedDur)
  detect change/1(change) -> params buffer/Trigger
  params buffer/2(pos) -> MATLAB Function/2(Pstart)
  pos/1 -> params buffer/2(pos_)
  vel/1 -> Terminator/1

== system FingerEAERCtrl/trajectory calculator/mode 2: auto initiated/rt minimum jerk trajectory1 ==
  note: tra jectory calculator for a single finger
  Pdes : Inport
  Tdes : Inport  Port=2
  pos : Inport  Port=3
  vel : Inport  Port=4
  MATLAB Function : MATLAB Function  TreatAsAtomicUnit=on
  Terminator : Terminator
  detect change : Subsystem
  params buffer : Subsystem
  trajectory : Outport
  wires:
  [TARGET_TIME] -> params buffer/4(t), MATLAB Function/5(t)
  Tdes/1 -> detect change/1(pDes), params buffer/3(tHit_)
  Pdes/1 -> params buffer/1(pDes_)
  params buffer/1(pDes) -> MATLAB Function/1(Pd)
  params buffer/3(tHit) -> MATLAB Function/3(th)
  params buffer/4(dur) -> MATLAB Function/4(dur)
  MATLAB Function/1(des) -> trajectory/1
  [FIXED_DUR] -> params buffer/5(fixedDur)
  detect change/1(change) -> params buffer/Trigger
  params buffer/2(pos) -> MATLAB Function/2(Pstart)
  pos/1 -> params buffer/2(pos_)
  vel/1 -> Terminator/1

== system FingerEAERCtrl/trajectory calculator/mode 3: auto init no return/rt minimum jerk trajectory ==
  note: trajectory calculator for a single finger
  Pdes : Inport
  Tdes : Inport  Port=2
  vel : Inport  Port=3
  MATLAB Function : MATLAB Function  TreatAsAtomicUnit=on
  Memory : Memory
  Memory1 : Memory
  Terminator : Terminator
  detect change : Subsystem
  params buffer : Subsystem
  trajectory : Outport
  wires:
  [TARGET_TIME] -> detect change/1(pDes), MATLAB Function/4(t)
  Tdes/1 -> params buffer/2(tHit_)
  Pdes/1 -> params buffer/1(pDes_)
  params buffer/1(pDes) -> MATLAB Function/1(Pd)
  params buffer/2(tHit) -> MATLAB Function/2(th)
  params buffer/3(dur) -> MATLAB Function/3(dur)
  MATLAB Function/1(des) -> trajectory/1
  [FIXED_DUR] -> params buffer/3(fixedDur)
  detect change/1(change) -> params buffer/Trigger
  vel/1 -> Terminator/1
  MATLAB Function/2(Phold) -> Memory/1
  Memory/1 -> MATLAB Function/5(Phold_)
  MATLAB Function/3(state) -> Memory1/1
  Memory1/1 -> MATLAB Function/6(state_)

== system FingerEAERCtrl/trajectory calculator/mode 3: auto init no return/rt minimum jerk trajectory1 ==
  note: trajectory calculator for a single finger
  Pdes : Inport
  Tdes : Inport  Port=2
  vel : Inport  Port=3
  MATLAB Function : MATLAB Function  TreatAsAtomicUnit=on
  Memory : Memory
  Memory1 : Memory
  Terminator : Terminator
  detect change : Subsystem
  params buffer : Subsystem
  trajectory : Outport
  wires:
  [TARGET_TIME] -> detect change/1(pDes), MATLAB Function/4(t)
  Tdes/1 -> params buffer/2(tHit_)
  Pdes/1 -> params buffer/1(pDes_)
  params buffer/1(pDes) -> MATLAB Function/1(Pd)
  params buffer/2(tHit) -> MATLAB Function/2(th)
  params buffer/3(dur) -> MATLAB Function/3(dur)
  MATLAB Function/1(des) -> trajectory/1
  [FIXED_DUR] -> params buffer/3(fixedDur)
  detect change/1(change) -> params buffer/Trigger
  vel/1 -> Terminator/1
  MATLAB Function/2(Phold) -> Memory/1
  Memory/1 -> MATLAB Function/5(Phold_)
  MATLAB Function/3(state) -> Memory1/1
  Memory1/1 -> MATLAB Function/6(state_)

== system FingerEAERCtrl/trajectory calculator/mode 4: sub init no return/get human force ==
  note: flip robot force to get human force
  forces : Inport
  Constant : Constant  Value=-1
  Demux3 : Demux  Outputs=2
  Product : Product  RndMeth=Zero
  Product1 : Product  RndMeth=Zero
  h_force1 : Outport
  h_force2 : Outport  Port=2
  wires:
  forces/1 -> Demux3/1
  Constant/1 -> Product1/2, Product/2
  Product/1 -> h_force1/1
  Demux3/1 -> Product/1
  Demux3/2 -> Product1/1
  Product1/1 -> h_force2/1

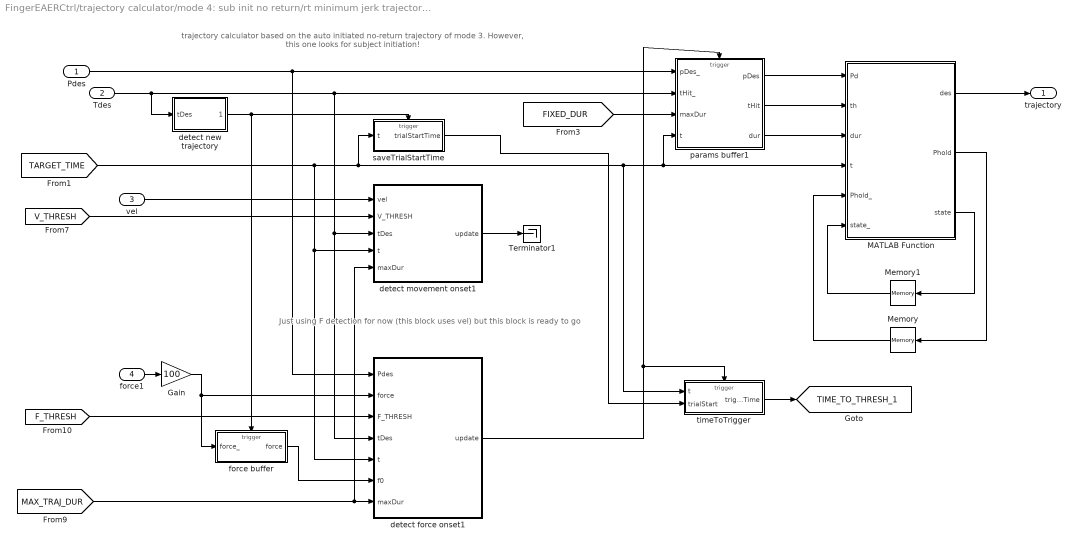
== system FingerEAERCtrl/trajectory calculator/mode 4: sub init no return/rt minimum jerk trajectory1 ==
  note: trajectory calculator based on the auto initiated no-return trajectory of mode 3.
      | However, this one looks for subject initiation!
  note: Just using F detection for now
      | (this block uses vel)
      | but this block is ready to go
  Pdes : Inport
  Tdes : Inport  Port=2
  vel : Inport  Port=3
  force1 : Inport  Port=4
  Gain : Gain  Gain=100
  MATLAB Function : MATLAB Function  TreatAsAtomicUnit=on
  Memory : Memory
  Memory1 : Memory
  Terminator1 : Terminator
  detect force onset1 : MATLAB Function  TreatAsAtomicUnit=on
  detect movement onset1 : MATLAB Function  TreatAsAtomicUnit=on
  detect new trajectory : Subsystem
  force buffer : Subsystem
  params buffer1 : Subsystem
  saveTrialStartTime : Subsystem
  timeToTrigger : Subsystem
  trajectory : Outport
  tag scope: TIME_TO_THRESH_1=global
  wires:
  Tdes/1 -> detect new trajectory/1(tDes), params buffer1/2(tHit_), detect force onset1/4(tDes), detect movement onset1/3(tDes)
  [V_THRESH] -> detect movement onset1/2(V_THRESH)
  [F_THRESH] -> detect force onset1/3(F_THRESH)
  [TARGET_TIME] -> saveTrialStartTime/1(t), timeToTrigger/1(t), params buffer1/4(t), MATLAB Function/4(t), detect force onset1/5(t), detect movement onset1/4(t)
  [MAX_TRAJ_DUR] -> detect movement onset1/5(maxDur), detect force onset1/7(maxDur)
  vel/1 -> detect movement onset1/1(vel)
  force1/1 -> Gain/1
  Pdes/1 -> detect force onset1/1(Pdes), params buffer1/1(pDes_)
  MATLAB Function/1(des) -> trajectory/1
  MATLAB Function/2(Phold) -> Memory/1
  Memory/1 -> MATLAB Function/5(Phold_)
  MATLAB Function/3(state) -> Memory1/1
  Memory1/1 -> MATLAB Function/6(state_)
  [FIXED_DUR] -> params buffer1/3(maxDur)
  params buffer1/1(pDes) -> MATLAB Function/1(Pd)
  params buffer1/2(tHit) -> MATLAB Function/2(th)
  params buffer1/3(dur) -> MATLAB Function/3(dur)
  detect movement onset1/1(update) -> Terminator1/1
  detect force onset1/1(update) -> timeToTrigger/Trigger, params buffer1/Trigger
  force buffer/1(force) -> detect force onset1/6(f0)
  detect new trajectory/1(change) -> force buffer/Trigger, saveTrialStartTime/Trigger
  Gain/1 -> detect force onset1/2(force), force buffer/1(force_)
  saveTrialStartTime/1(trialStartTime) -> timeToTrigger/2(trialStart)
  timeToTrigger/1(triggerTime) -> [TIME_TO_THRESH_1]

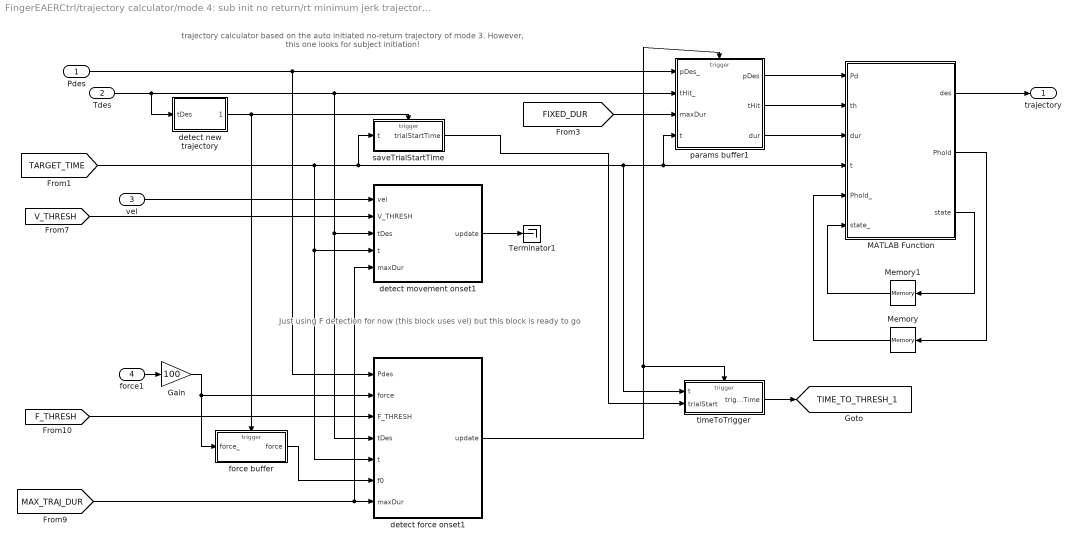
== system FingerEAERCtrl/trajectory calculator/mode 4: sub init no return/rt minimum jerk trajectory2 ==
  note: trajectory calculator based on the auto initiated no-return trajectory of mode 3.
      | However, this one looks for subject initiation!
  note: Just using F detection for now
      | (this block uses vel)
      | but this block is ready to go
  Pdes : Inport
  Tdes : Inport  Port=2
  vel : Inport  Port=3
  force1 : Inport  Port=4
  Gain : Gain  Gain=100
  MATLAB Function : MATLAB Function  TreatAsAtomicUnit=on
  Memory : Memory
  Memory1 : Memory
  Terminator1 : Terminator
  detect force onset1 : MATLAB Function  TreatAsAtomicUnit=on
  detect movement onset1 : MATLAB Function  TreatAsAtomicUnit=on
  detect new trajectory : Subsystem
  force buffer : Subsystem
  params buffer1 : Subsystem
  saveTrialStartTime : Subsystem
  timeToTrigger : Subsystem
  trajectory : Outport
  tag scope: TIME_TO_THRESH_1=global
  wires:
  Tdes/1 -> detect new trajectory/1(tDes), params buffer1/2(tHit_), detect force onset1/4(tDes), detect movement onset1/3(tDes)
  [V_THRESH] -> detect movement onset1/2(V_THRESH)
  [F_THRESH] -> detect force onset1/3(F_THRESH)
  [TARGET_TIME] -> saveTrialStartTime/1(t), timeToTrigger/1(t), params buffer1/4(t), MATLAB Function/4(t), detect force onset1/5(t), detect movement onset1/4(t)
  [MAX_TRAJ_DUR] -> detect movement onset1/5(maxDur), detect force onset1/7(maxDur)
  vel/1 -> detect movement onset1/1(vel)
  force1/1 -> Gain/1
  Pdes/1 -> detect force onset1/1(Pdes), params buffer1/1(pDes_)
  MATLAB Function/1(des) -> trajectory/1
  MATLAB Function/2(Phold) -> Memory/1
  Memory/1 -> MATLAB Function/5(Phold_)
  MATLAB Function/3(state) -> Memory1/1
  Memory1/1 -> MATLAB Function/6(state_)
  [FIXED_DUR] -> params buffer1/3(maxDur)
  params buffer1/1(pDes) -> MATLAB Function/1(Pd)
  params buffer1/2(tHit) -> MATLAB Function/2(th)
  params buffer1/3(dur) -> MATLAB Function/3(dur)
  detect movement onset1/1(update) -> Terminator1/1
  detect force onset1/1(update) -> timeToTrigger/Trigger, params buffer1/Trigger
  force buffer/1(force) -> detect force onset1/6(f0)
  detect new trajectory/1(change) -> force buffer/Trigger, saveTrialStartTime/Trigger
  Gain/1 -> detect force onset1/2(force), force buffer/1(force_)
  saveTrialStartTime/1(trialStartTime) -> timeToTrigger/2(trialStart)
  timeToTrigger/1(triggerTime) -> [TIME_TO_THRESH_1]

== system FingerEAERCtrl/trajectory calculator/mode 1: sub-init/rt minimum jerk trajectory calc/params buffer ==
  pDes_ : Inport
  tHit_ : Inport  Port=2
  t : Inport  Port=3
  Trigger : TriggerPort  PortDimensions=1
  buffer the trajectory params : MATLAB Function  TreatAsAtomicUnit=on
  pDes : Outport
  tHit : Outport  Port=2
  dur : Outport  Port=3
  wires:
  pDes_/1 -> buffer the trajectory params/1(pDes_)
  buffer the trajectory params/1(pDes) -> pDes/1
  t/1 -> buffer the trajectory params/3(t)
  buffer the trajectory params/2(tHit) -> tHit/1
  tHit_/1 -> buffer the trajectory params/2(tHit_)
  buffer the trajectory params/3(dur) -> dur/1

== system FingerEAERCtrl/trajectory calculator/mode 1: sub-init/rt minimum jerk trajectory calc1/params buffer ==
  pDes_ : Inport
  tHit_ : Inport  Port=2
  t : Inport  Port=3
  Trigger : TriggerPort  PortDimensions=1
  buffer the trajectory params : MATLAB Function  TreatAsAtomicUnit=on
  pDes : Outport
  tHit : Outport  Port=2
  dur : Outport  Port=3
  wires:
  pDes_/1 -> buffer the trajectory params/1(pDes_)
  buffer the trajectory params/1(pDes) -> pDes/1
  t/1 -> buffer the trajectory params/3(t)
  buffer the trajectory params/2(tHit) -> tHit/1
  tHit_/1 -> buffer the trajectory params/2(tHit_)
  buffer the trajectory params/3(dur) -> dur/1

== system FingerEAERCtrl/trajectory calculator/mode 2: auto initiated/rt minimum jerk trajectory/detect change ==
  note: I added this block that that we can switch between subject initiated movements and robot initiated movements
  pDes : Inport
  MATLAB Function1 : MATLAB Function  TreatAsAtomicUnit=on
  Memory1 : Memory
  change : Outport
  wires:
  pDes/1 -> MATLAB Function1/1(pDes)
  Memory1/1 -> MATLAB Function1/2(pDes_)
  MATLAB Function1/1(change) -> change/1, Memory1/1

== system FingerEAERCtrl/trajectory calculator/mode 2: auto initiated/rt minimum jerk trajectory/params buffer ==
  pDes_ : Inport
  pos_ : Inport  Port=2
  tHit_ : Inport  Port=3
  t : Inport  Port=4
  fixedDur : Inport  Port=5
  Trigger : TriggerPort  PortDimensions=1
  buffer the trajectory params : MATLAB Function  TreatAsAtomicUnit=on
  pDes : Outport
  pos : Outport  Port=2
  tHit : Outport  Port=3
  dur : Outport  Port=4
  wires:
  pDes_/1 -> buffer the trajectory params/1(pDes_)
  buffer the trajectory params/1(pDes) -> pDes/1
  t/1 -> buffer the trajectory params/4(t)
  buffer the trajectory params/3(tHit) -> tHit/1
  tHit_/1 -> buffer the trajectory params/3(tHit_)
  fixedDur/1 -> dur/1
  pos_/1 -> buffer the trajectory params/2(pos_)
  buffer the trajectory params/2(pos) -> pos/1

== system FingerEAERCtrl/trajectory calculator/mode 2: auto initiated/rt minimum jerk trajectory1/detect change ==
  note: I added this block that that we can switch between subject initiated movements and robot initiated movements
  pDes : Inport
  MATLAB Function1 : MATLAB Function  TreatAsAtomicUnit=on
  Memory1 : Memory
  change : Outport
  wires:
  pDes/1 -> MATLAB Function1/1(pDes)
  Memory1/1 -> MATLAB Function1/2(pDes_)
  MATLAB Function1/1(change) -> change/1, Memory1/1

== system FingerEAERCtrl/trajectory calculator/mode 2: auto initiated/rt minimum jerk trajectory1/params buffer ==
  pDes_ : Inport
  pos_ : Inport  Port=2
  tHit_ : Inport  Port=3
  t : Inport  Port=4
  fixedDur : Inport  Port=5
  Trigger : TriggerPort  PortDimensions=1
  buffer the trajectory params : MATLAB Function  TreatAsAtomicUnit=on
  pDes : Outport
  pos : Outport  Port=2
  tHit : Outport  Port=3
  dur : Outport  Port=4
  wires:
  pDes_/1 -> buffer the trajectory params/1(pDes_)
  buffer the trajectory params/1(pDes) -> pDes/1
  t/1 -> buffer the trajectory params/4(t)
  buffer the trajectory params/3(tHit) -> tHit/1
  tHit_/1 -> buffer the trajectory params/3(tHit_)
  fixedDur/1 -> dur/1
  pos_/1 -> buffer the trajectory params/2(pos_)
  buffer the trajectory params/2(pos) -> pos/1

== system FingerEAERCtrl/trajectory calculator/mode 3: auto init no return/rt minimum jerk trajectory/detect change ==
  note: I added this block that that we can switch between subject initiated movements and robot initiated movements
  pDes : Inport
  MATLAB Function1 : MATLAB Function  TreatAsAtomicUnit=on
  Memory1 : Memory
  change : Outport
  wires:
  pDes/1 -> MATLAB Function1/1(pDes)
  Memory1/1 -> MATLAB Function1/2(pDes_)
  MATLAB Function1/1(change) -> change/1, Memory1/1

== system FingerEAERCtrl/trajectory calculator/mode 3: auto init no return/rt minimum jerk trajectory/params buffer ==
  pDes_ : Inport
  tHit_ : Inport  Port=2
  fixedDur : Inport  Port=3
  Trigger : TriggerPort  PortDimensions=1
  buffer the trajectory params : MATLAB Function  TreatAsAtomicUnit=on
  pDes : Outport
  tHit : Outport  Port=2
  dur : Outport  Port=3
  wires:
  pDes_/1 -> buffer the trajectory params/1(pDes_)
  buffer the trajectory params/1(pDes) -> pDes/1
  buffer the trajectory params/2(tHit) -> tHit/1
  tHit_/1 -> buffer the trajectory params/2(tHit_)
  fixedDur/1 -> dur/1

== system FingerEAERCtrl/trajectory calculator/mode 3: auto init no return/rt minimum jerk trajectory1/detect change ==
  note: I added this block that that we can switch between subject initiated movements and robot initiated movements
  pDes : Inport
  MATLAB Function1 : MATLAB Function  TreatAsAtomicUnit=on
  Memory1 : Memory
  change : Outport
  wires:
  pDes/1 -> MATLAB Function1/1(pDes)
  Memory1/1 -> MATLAB Function1/2(pDes_)
  MATLAB Function1/1(change) -> change/1, Memory1/1

== system FingerEAERCtrl/trajectory calculator/mode 3: auto init no return/rt minimum jerk trajectory1/params buffer ==
  pDes_ : Inport
  tHit_ : Inport  Port=2
  fixedDur : Inport  Port=3
  Trigger : TriggerPort  PortDimensions=1
  buffer the trajectory params : MATLAB Function  TreatAsAtomicUnit=on
  pDes : Outport
  tHit : Outport  Port=2
  dur : Outport  Port=3
  wires:
  pDes_/1 -> buffer the trajectory params/1(pDes_)
  buffer the trajectory params/1(pDes) -> pDes/1
  buffer the trajectory params/2(tHit) -> tHit/1
  tHit_/1 -> buffer the trajectory params/2(tHit_)
  fixedDur/1 -> dur/1

== system FingerEAERCtrl/trajectory calculator/mode 4: sub init no return/rt minimum jerk trajectory1/detect new trajectory ==
  note: detects when tDes is changed, and trips the trigger
  tDes : Inport
  MATLAB Function1 : MATLAB Function  TreatAsAtomicUnit=on
  Memory2 : Memory
  change : Outport
  wires:
  tDes/1 -> MATLAB Function1/1(tDes)
  MATLAB Function1/1(change) -> change/1
  MATLAB Function1/2(tDesOut) -> Memory2/1
  Memory2/1 -> MATLAB Function1/2(tDesLast)

== system FingerEAERCtrl/trajectory calculator/mode 4: sub init no return/rt minimum jerk trajectory1/force buffer ==
  force_ : Inport
  Trigger : TriggerPort  PortDimensions=1
  buffer the initial force value : MATLAB Function  TreatAsAtomicUnit=on
  force : Outport
  wires:
  force_/1 -> buffer the initial force value/1(force_)
  buffer the initial force value/1(force) -> force/1
